simulink library "magnetometerSensorHW_sl"  (R2024b)
settings: Solver=VariableStepAuto  StartTime=0.0  StopTime=10.0  RelTol=1e-3
undefined symbols (not defined in the file): magError, magErrorFlag
settings Model: Creator=gilbu
settings RTWCC: GPUComputeCapability=3.5

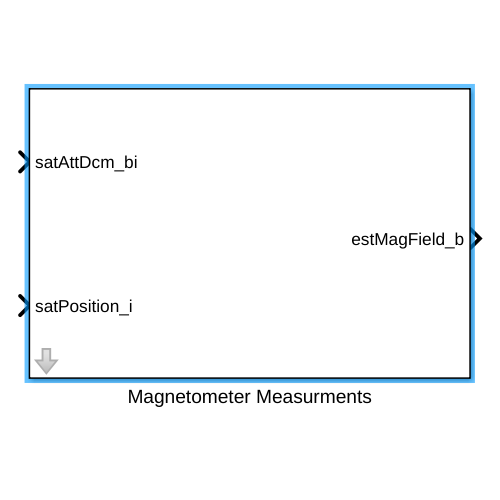
[thumbnail: Simulink's stored preview of the top-level diagram]
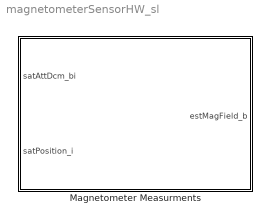
== system magnetometerSensorHW_sl ==
  Magnetometer Measurments : Subsystem  mask{magErrorFlag=magErrorFlag, magError=magError}
      mask prompts: magErrorFlag "Magnetometer Error Flag <1> [-]"; magError "Sensor Error<3> [nT]"
      mask DialogControl DescTextVar Prompt: Simulated magnetometer HW for attitude measurements. Error includes constant 3-axis error. Errors can be tured on an off using magErrorFlag and parameters.
      mask DialogControl Control2 Prompt: Magnetometer Error Flag equal to one will allow error into the attitude measurements

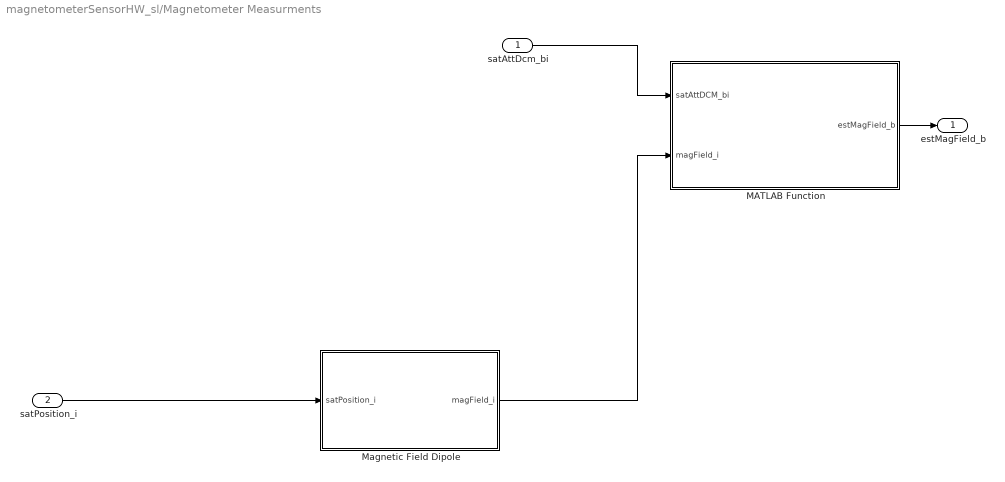
== system magnetometerSensorHW_sl/Magnetometer Measurments ==
  satAttDcm_bi : Inport
  satPosition_i : Inport  Port=2
  MATLAB Function : MATLAB Function  TreatAsAtomicUnit=on
  Magnetic Field Dipole : MATLAB Function  TreatAsAtomicUnit=on
  estMagField_b : Outport
  wires:
  satAttDcm_bi/1 -> MATLAB Function/1(satAttDCM_bi)
  MATLAB Function/1(estMagField_b) -> estMagField_b/1
  Magnetic Field Dipole/1(magField_i) -> MATLAB Function/2(magField_i)
  satPosition_i/1 -> Magnetic Field Dipole/1(satPosition_i)

== matlab function magnetometerSensorHW_sl/Magnetometer Measurments/MATLAB Function ==
  data: satAttDCM_bi input double size=3,3; magField_i input size=3; estMagField_b output size=3; magError parameter size=3
% Author: Antonio Gil Buitrago
function estMagField_b = magnetometerMeasurement( ...
    satAttDCM_bi,magField_i,... %inputs
   magError... % Parameters
    )
%-------------------------------------------------------------------------------
% Simulated Noise Measurement

estMagField_b = satAttDCM_bi*magField_i + magError;


%-------------------------------------------------------------------------------
end

== matlab function magnetometerSensorHW_sl/Magnetometer Measurments/Magnetic Field Dipole ==
  data: satPosition_i input; magField_i output
% Author: Antonio Gil Buitrago
function magField_i = magFieldDipole( ...
    satPosition_i)
%-------------------------------------------------------------------------------
% Initialize Variables
x = satPosition_i(1);
y = satPosition_i(2);
z = satPosition_i(3);
r = norm(satPosition_i);

% Magnetic Moment
M = 8.22e22;
%-------------------------------------------------------------------------------
% Magnetic Field Strength

B_X = 3*M*x*z/r^5;

B_Y = 3*M*y*z/r^5;

B_Z = M*(3*z^2-r^2)/r^5;

magField_i = [B_X ; B_Y; B_Z];

%-------------------------------------------------------------------------------
end
